simulink model "LMI_lema_5_statefeedback_robusto"  (Simulink 7.7)
settings: Solver=ode45  StartTime=0.0  StopTime=1900  RelTol=1e-3
values from neighbouring files (symbols this model uses):
  QT =     [FaseMinima.mat]    (also in FaseNaoMinima.mat; FaseNaoMinimaMudandoApenasGama.mat; settup.m = dynamics())
settings Model: Creator=Arthur  LastModifiedBy=Arthur
settings DebuggingCC: UnderspecifiedInitializationDetection=Simplified

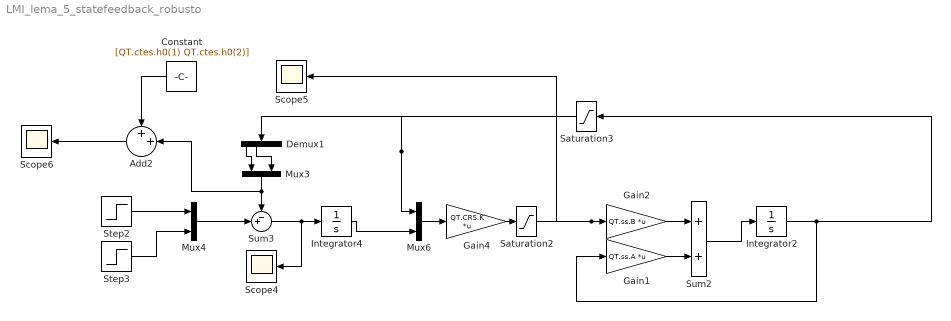
== system LMI_lema_5_statefeedback_robusto ==
  Add2 : Sum  Inputs=++|
  Constant : Constant  Value=[QT.ctes.h0(1) QT.ctes.h0(2)]
  Demux1 : Demux
  Gain1 : Gain  Gain=QT.ss.A  Multiplication=Matrix(K*u)
  Gain2 : Gain  Gain=QT.ss.B  Multiplication=Matrix(K*u)
  Gain4 : Gain  Gain=QT.CR5.K  Multiplication=Matrix(K*u)
  Integrator2 : Integrator
  Integrator4 : Integrator
  Mux3 : Mux  Inputs=2
  Mux4 : Mux  Inputs=2
  Mux6 : Mux  Inputs=2
  Saturation2 : Saturate  UpperLimit=1.5  LowerLimit=-1.5
  Saturation3 : Saturate  UpperLimit=10  LowerLimit=-5
  Scope4 : Scope
      settings: YMin=-0.75  YMax=2.25  SaveName=ScopeData3  SampleTime=1
  Scope5 : Scope
      settings: YMin=-0.75  YMax=2.25  SaveName=ScopeData4  SampleInput=on  SampleTime=1
  Scope6 : Scope
      settings: TimeRange=10  SaveName=Simulado
  Step2 : Step  Time=300  SampleTime=0
  Step3 : Step  Time=1100  SampleTime=0
  Sum2 : Sum
  Sum3 : Sum  Inputs=-+|
  wires:
  Gain1/1 -> Sum2/2
  Gain2/1 -> Sum2/1
  Step2/1 -> Mux4/1
  Step3/1 -> Mux4/2
  Integrator2/1 -> Gain1/1, Saturation3/1
  Sum2/1 -> Integrator2/1
  Gain4/1 -> Saturation2/1
  Mux6/1 -> Gain4/1
  Integrator4/1 -> Mux6/2
  Sum3/1 -> Integrator4/1, Scope4/1
  Mux4/1 -> Sum3/2
  Demux1/1 -> Mux3/1
  Demux1/2 -> Mux3/2
  Mux3/1 -> Sum3/1, Add2/2
  Saturation2/1 -> Gain2/1, Scope5/1
  Saturation3/1 -> Mux6/1, Demux1/1
  Add2/1 -> Scope6/1
  Constant/1 -> Add2/1
